simulink model "computed_torque_controller"  (R2020a)
settings: Solver=VariableStepAuto  StartTime=0.0  StopTime=50  RelTol=1e-3
model workspace (MAT data in the model file):
  kd = 0
  kp = 0
libraries: aerolibutil x4, sharedutil x2, simulink x1
settings Model: Creator=Sebas  LastModifiedBy=Sebas
settings SolverCC: ZeroCrossAlgorithm=Adaptive
settings DebuggingCC: MaskedZcDiagnostic=none  IgnoredZcDiagnostic=none

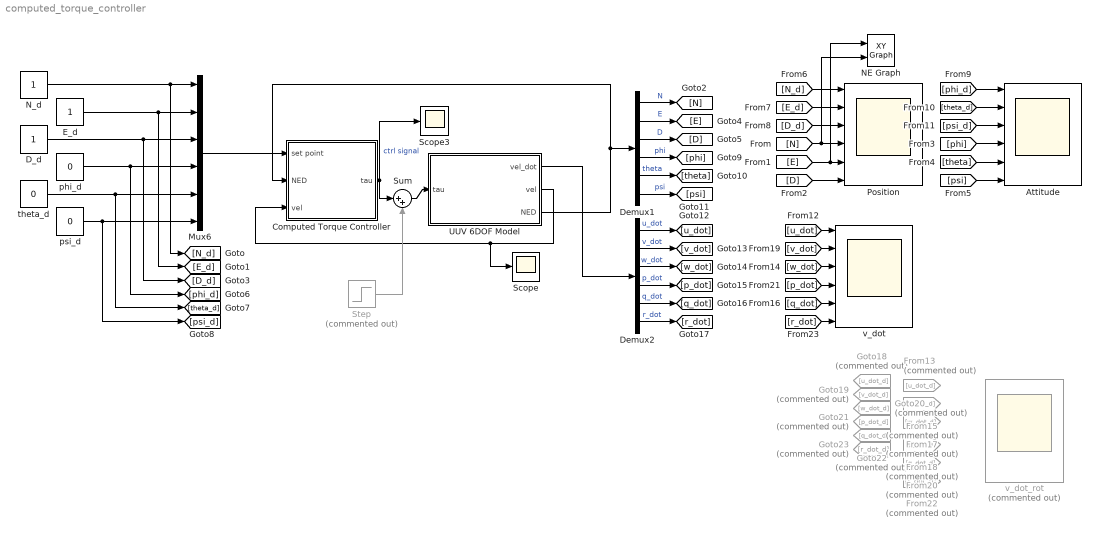
== system computed_torque_controller ==
  Attitude : Scope  NumInputPorts=6
  Computed Torque Controller : Subsystem
  D_d : Constant
  Demux1 : Demux  Outputs=6
  Demux2 : Demux  Outputs=6
  E_d : Constant
  From13 : From  Commented=on  GotoTag=u_dot_d
  From15 : From  Commented=on  GotoTag=v_dot_d
  From17 : From  Commented=on  GotoTag=w_dot_d
  From18 : From  Commented=on  GotoTag=p_dot_d
  From20 : From  Commented=on  GotoTag=q_dot_d
  From22 : From  Commented=on  GotoTag=r_dot_d
  Goto18 : Goto  Commented=on  GotoTag=u_dot_d
  Goto19 : Goto  Commented=on  GotoTag=v_dot_d
  Goto20 : Goto  Commented=on  GotoTag=w_dot_d
  Goto21 : Goto  Commented=on  GotoTag=p_dot_d
  Goto22 : Goto  Commented=on  GotoTag=q_dot_d
  Goto23 : Goto  Commented=on  GotoTag=r_dot_d
  Mux6 : Mux  Inputs=6
  NE Graph : simulink/Sinks/XY Graph  xmin=-1  xmax=5  ymin=-1  ymax=2  st=-1
  N_d : Constant
  Position : Scope  NumInputPorts=6
  Scope : Scope
  Scope3 : Scope
  Step : Step  Commented=on  Time=20  After=[30;30;30;5;5;5]  SampleTime=0
  Sum : Sum  Inputs=|++
  UUV 6DOF Model : Subsystem
  phi_d : Constant  Value=0
  psi_d : Constant  Value=0
  theta_d : Constant  Value=0
  v_dot : Scope  NumInputPorts=6
  v_dot_rot : Scope  Commented=on  NumInputPorts=6
  wires:
  UUV 6DOF Model/3(NED) -> Computed Torque Controller/2(NED), Demux1/1
  [N_d] -> Position/1
  [E_d] -> Position/2
  [D_d] -> Position/3
  [N] -> Position/4, NE Graph/2
  [D] -> Position/6
  [E] -> Position/5, NE Graph/1
  Demux1/1 -> [N]  "N"
  Demux1/2 -> [E]  "E"
  Demux1/3 -> [D]  "D"
  [phi_d] -> Attitude/1
  [phi] -> Attitude/4
  [psi_d] -> Attitude/3
  [theta] -> Attitude/5
  [psi] -> Attitude/6
  [theta_d] -> Attitude/2
  Demux1/4 -> [phi]  "phi"
  Demux1/5 -> [theta]  "theta"
  Demux1/6 -> [psi]  "psi"
  UUV 6DOF Model/2(vel) -> Computed Torque Controller/3(vel), Scope/1
  UUV 6DOF Model/1(vel_dot) -> Demux2/1
  [u_dot] -> v_dot/1
  [v_dot] -> v_dot/2
  [w_dot] -> v_dot/3
  [p_dot] -> v_dot/4
  [q_dot] -> v_dot/5
  [r_dot] -> v_dot/6
  Demux2/1 -> [u_dot]  "u_dot"
  Demux2/5 -> [q_dot]  "q_dot"
  Demux2/3 -> [w_dot]  "w_dot"
  Demux2/6 -> [r_dot]  "r_dot"
  Demux2/4 -> [p_dot]  "p_dot"
  Demux2/2 -> [v_dot]  "v_dot"
  D_d/1 -> Mux6/3, [D_d]
  theta_d/1 -> [theta_d], Mux6/5
  Mux6/1 -> Computed Torque Controller/1(set point)
  phi_d/1 -> Mux6/4, [phi_d]
  E_d/1 -> [E_d], Mux6/2
  N_d/1 -> [N_d], Mux6/1
  psi_d/1 -> [psi_d], Mux6/6
  Step/1 -> Sum/2
  Computed Torque Controller/1(tau) -> Sum/1, Scope3/1  "ctrl signal"
  Sum/1 -> UUV 6DOF Model/1(tau)

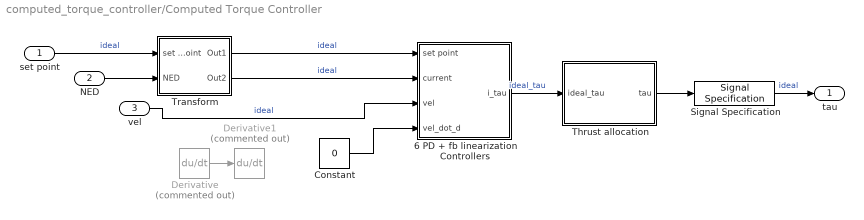
== system computed_torque_controller/Computed Torque Controller ==
  set point : Inport
  NED : Inport  Port=2
  vel : Inport  Port=3
  6 PD + fb linearization Controllers : Subsystem  mask(6 Degrees-of-freedom P-D Controller){surge_kd=0.35, surge_kp=0.7, sway_kd=0.7, sway_kp=0.6, heave_kd=0.2, heave_kp=0.7, roll_kd=1.3, roll_kp=10, pitch_kd=0.05, pitch_kp=0.2, yaw_kd=1.2, yaw_kp=3}
      mask prompts: surge_kd "Surge K derivative"; surge_kp "Surge K proportional"; sway_kd "Sway K derivative"; sway_kp "Sway K proportional"; heave_kd "Heave K derivative"; heave_kp "Heave K proportional"; roll_kd "Roll K derivative"; roll_kp "Roll K proportional"; pitch_kd "Pitch K derivative"; pitch_kp "Pitch K proportional"; yaw_kd "Yaw K derivative"; yaw_kp "Yaw K proportional"
      mask help: Implementation of 6 PD controllers for each degree of freedom
      mask DialogControl ParameterGroupVar Prompt: Gains
  Constant : Constant  Value=0
  Derivative : Derivative  Commented=on
  Derivative1 : Derivative  Commented=on
  Signal Specification : SignalSpecification  Dimensions=6
  Thrust allocation : Subsystem
  Transform : Subsystem
  tau : Outport
  wires:
  Transform/1(Out1) -> 6 PD + fb linearization Controllers/1(set point)  "ideal"
  NED/1 -> Transform/2(NED)
  Signal Specification/1 -> tau/1  "ideal"
  Transform/2(Out2) -> 6 PD + fb linearization Controllers/2(current)  "ideal"
  Thrust allocation/1(tau) -> Signal Specification/1
  6 PD + fb linearization Controllers/1(i_tau) -> Thrust allocation/1(ideal_tau)  "ideal_tau"
  vel/1 -> 6 PD + fb linearization Controllers/3(vel)  "ideal"
  set point/1 -> Transform/1(set point)  "ideal"
  Constant/1 -> 6 PD + fb linearization Controllers/4(vel_dot_d)
  Derivative/1 -> Derivative1/1

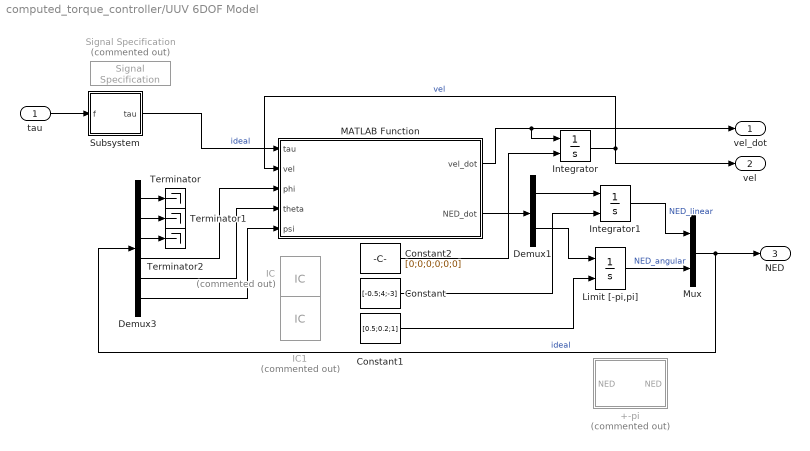
== system computed_torque_controller/UUV 6DOF Model ==
  tau : Inport
  +-pi : MATLAB Function  Commented=on  TreatAsAtomicUnit=on
  Constant : Constant  Value=[-0.5;4;-3]
  Constant1 : Constant  Value=[0.5;0.2;1]
  Constant2 : Constant  Value=[0;0;0;0;0;0]
  Demux1 : Demux  Outputs=2
  Demux3 : Demux  Outputs=6
  IC : InitialCondition  Commented=on  Value=[0;0;0;0;0;0]
  IC1 : InitialCondition  Commented=on  Value=[1;1;1;1;1;1]
  Integrator : Integrator  InitialConditionSource=external
  Integrator1 : Integrator  InitialConditionSource=external
  Limit [-pi,pi] : Integrator  InitialConditionSource=external  WrapState=on
  MATLAB Function : MATLAB Function  TreatAsAtomicUnit=on
  Mux : Mux  Inputs=2
  Signal Specification : SignalSpecification  Commented=on  Dimensions=6
  Subsystem : Subsystem
  Terminator : Terminator
  Terminator1 : Terminator
  Terminator2 : Terminator
  vel_dot : Outport
  vel : Outport  Port=2
  NED : Outport  Port=3
  wires:
  Constant/1 -> Integrator1/2
  Constant1/1 -> Limit [-pi,pi]/2
  Constant2/1 -> Integrator/2
  MATLAB Function/2(NED_dot) -> Demux1/1
  Demux1/1 -> Integrator1/1
  Demux1/2 -> Limit [-pi,pi]/1
  Limit [-pi,pi]/1 -> Mux/2  "NED_angular"
  tau/1 -> Subsystem/1(f)
  Subsystem/1(tau) -> MATLAB Function/1(tau)  "ideal"
  Demux3/3 -> Terminator2/1
  Demux3/1 -> Terminator/1
  Demux3/2 -> Terminator1/1
  Integrator1/1 -> Mux/1  "NED_linear"
  Demux3/6 -> MATLAB Function/5(psi)
  Demux3/5 -> MATLAB Function/4(theta)
  Demux3/4 -> MATLAB Function/3(phi)
  Integrator/1 -> MATLAB Function/2(vel), vel/1  "vel"
  MATLAB Function/1(vel_dot) -> Integrator/1, vel_dot/1
  Mux/1 -> NED/1, Demux3/1  "ideal"

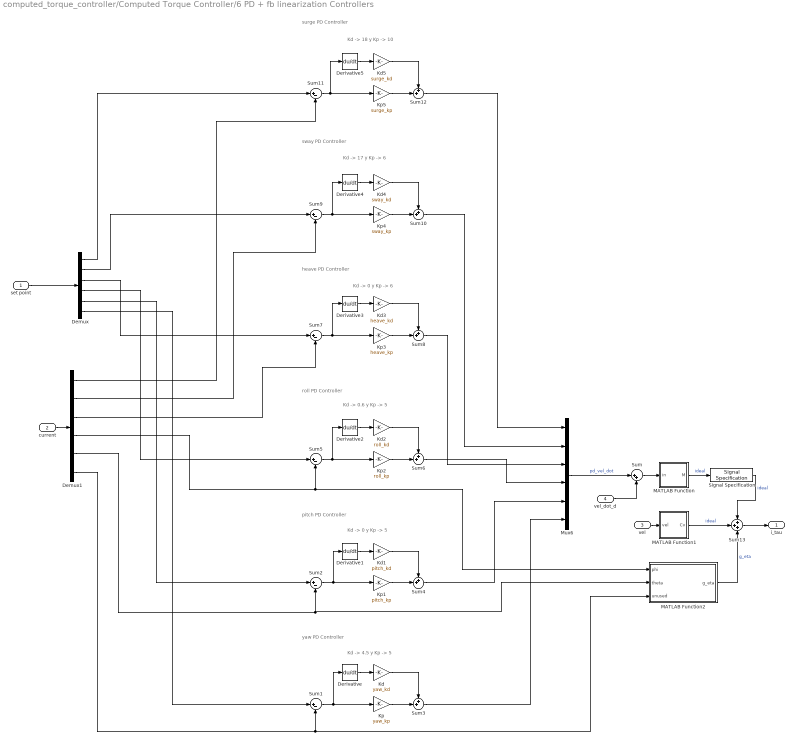
== system computed_torque_controller/Computed Torque Controller/6 PD + fb linearization Controllers ==
  note: surge PD Controller
  note: sway PD Controller
  note: heave PD Controller
  note: roll PD Controller
  note: pitch PD Controller
  note: yaw PD Controller
  note: Kd -> 4.5 y Kp -> 5
  note: Kd -> 0 y Kp -> 5
  note: Kd -> 0.6 y Kp -> 5
  note: Kd -> 0 y Kp -> 6
  note: Kd -> 17 y Kp -> 6
  note: Kd -> 18 y Kp -> 10
  set point : Inport
  current : Inport  Port=2
  vel : Inport  Port=3
  vel_dot_d : Inport  Port=4
  Demux : Demux  Outputs=6
  Demux1 : Demux  Outputs=6
  Derivative{,1..5} (6 alike) : Derivative
  Kd : Gain  Gain=yaw_kd
  Kd1 : Gain  Gain=pitch_kd
  Kd2 : Gain  Gain=roll_kd
  Kd3 : Gain  Gain=heave_kd
  Kd4 : Gain  Gain=sway_kd
  Kd5 : Gain  Gain=surge_kd
  Kp : Gain  Gain=yaw_kp
  Kp1 : Gain  Gain=pitch_kp
  Kp2 : Gain  Gain=roll_kp
  Kp3 : Gain  Gain=heave_kp
  Kp4 : Gain  Gain=sway_kp
  Kp5 : Gain  Gain=surge_kp
  MATLAB Function : MATLAB Function  TreatAsAtomicUnit=on
  MATLAB Function1 : MATLAB Function  TreatAsAtomicUnit=on
  MATLAB Function2 : MATLAB Function  TreatAsAtomicUnit=on
  Mux6 : Mux  Inputs=6
  Signal Specification : SignalSpecification  Dimensions=6
  Sum : Sum  Inputs=|++
  Sum{1..2,5,7,9,11} (6 alike) : Sum  Inputs=|+-
  Sum{3..4,6,8,10,12} (6 alike) : Sum  Inputs=++|
  Sum13 : Sum  Inputs=+++
  i_tau : Outport
  wires:
  Sum8/1 -> Mux6/3
  Sum4/1 -> Mux6/5
  Sum6/1 -> Mux6/4
  Sum3/1 -> Mux6/6
  Sum12/1 -> Mux6/1
  Sum10/1 -> Mux6/2
  Derivative/1 -> Kd/1
  Kp/1 -> Sum3/2
  Kd/1 -> Sum3/1
  Sum1/1 -> Derivative/1, Kp/1
  Sum2/1 -> Kp1/1, Derivative1/1
  Kd1/1 -> Sum4/1
  Kp1/1 -> Sum4/2
  Derivative1/1 -> Kd1/1
  Derivative2/1 -> Kd2/1
  Kp2/1 -> Sum6/2
  Kd2/1 -> Sum6/1
  Sum5/1 -> Derivative2/1, Kp2/1
  Derivative3/1 -> Kd3/1
  Kp3/1 -> Sum8/2
  Kd3/1 -> Sum8/1
  Sum7/1 -> Derivative3/1, Kp3/1
  Derivative4/1 -> Kd4/1
  Kp4/1 -> Sum10/2
  Kd4/1 -> Sum10/1
  Sum9/1 -> Derivative4/1, Kp4/1
  Derivative5/1 -> Kd5/1
  Kp5/1 -> Sum12/2
  Kd5/1 -> Sum12/1
  Sum11/1 -> Derivative5/1, Kp5/1
  current/1 -> Demux1/1
  Demux1/1 -> Sum11/2
  set point/1 -> Demux/1
  Demux/1 -> Sum11/1
  Demux/2 -> Sum9/1
  Demux1/2 -> Sum9/2
  Demux/3 -> Sum7/1
  Demux1/3 -> Sum7/2
  Demux/4 -> Sum5/1
  Demux1/4 -> MATLAB Function2/1(phi), Sum5/2
  Demux/5 -> Sum2/1
  Demux1/5 -> MATLAB Function2/2(theta), Sum2/2
  Demux/6 -> Sum1/1
  Demux1/6 -> MATLAB Function2/3(unused), Sum1/2
  Mux6/1 -> Sum/1  "pd_vel_dot"
  Sum/1 -> MATLAB Function/1(in)
  vel_dot_d/1 -> Sum/2
  Sum13/1 -> i_tau/1
  vel/1 -> MATLAB Function1/1(vel)
  MATLAB Function/1(M) -> Signal Specification/1  "ideal"
  MATLAB Function2/1(g_eta) -> Sum13/3  "g_eta"
  MATLAB Function1/1(Cv) -> Sum13/2  "ideal"
  Signal Specification/1 -> Sum13/1  "ideal"

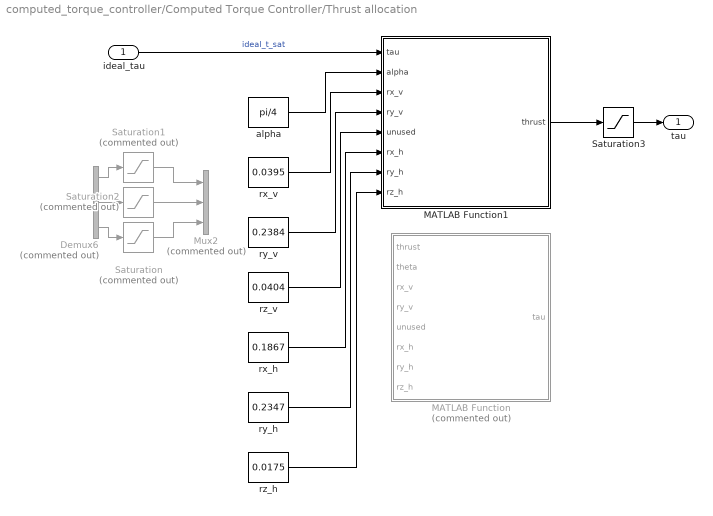
== system computed_torque_controller/Computed Torque Controller/Thrust allocation ==
  ideal_tau : Inport
  Demux6 : Demux  Commented=on  Outputs=3
  MATLAB Function : MATLAB Function  Commented=on  TreatAsAtomicUnit=on
  MATLAB Function1 : MATLAB Function  TreatAsAtomicUnit=on
  Mux2 : Mux  Commented=on  Inputs=3
  Saturation : Saturate  Commented=on  UpperLimit=70  LowerLimit=-70
  Saturation1 : Saturate  Commented=on  UpperLimit=100  LowerLimit=-100
  Saturation2 : Saturate  Commented=on  UpperLimit=100  LowerLimit=-100
  Saturation3 : Saturate  UpperLimit=35  LowerLimit=-35
  alpha : Constant  Value=pi/4
  rx_h : Constant  Value=0.1867
  rx_v : Constant  Value=0.0395
  ry_h : Constant  Value=0.2347
  ry_v : Constant  Value=0.2384
  rz_h : Constant  Value=0.0175
  rz_v : Constant  Value=0.0404
  tau : Outport
  wires:
  ideal_tau/1 -> MATLAB Function1/1(tau)  "ideal_t_sat"
  MATLAB Function1/1(thrust) -> Saturation3/1
  Saturation3/1 -> tau/1
  rx_v/1 -> MATLAB Function1/3(rx_v)
  alpha/1 -> MATLAB Function1/2(alpha)
  rx_h/1 -> MATLAB Function1/6(rx_h)
  ry_h/1 -> MATLAB Function1/7(ry_h)
  rz_h/1 -> MATLAB Function1/8(rz_h)
  ry_v/1 -> MATLAB Function1/4(ry_v)
  rz_v/1 -> MATLAB Function1/5(unused)
  Demux6/2 -> Saturation2/1
  Demux6/3 -> Saturation/1
  Saturation1/1 -> Mux2/1
  Saturation/1 -> Mux2/3
  Demux6/1 -> Saturation1/1
  Saturation2/1 -> Mux2/2

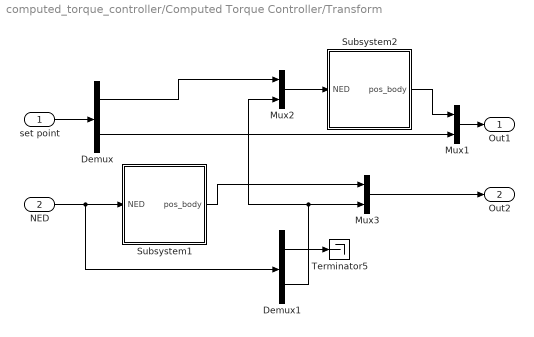
== system computed_torque_controller/Computed Torque Controller/Transform ==
  set point : Inport
  NED : Inport  Port=2
  Demux : Demux  Outputs=2
  Demux1 : Demux  Outputs=2
  Mux1 : Mux  Inputs=2
  Mux2 : Mux  Inputs=2
  Mux3 : Mux  Inputs=2
  Subsystem1 : Subsystem
  Subsystem2 : Subsystem
  Terminator5 : Terminator
  Out1 : Outport
  Out2 : Outport  Port=2
  wires:
  Demux/1 -> Mux2/1
  NED/1 -> Demux1/1, Subsystem1/1(NED)
  set point/1 -> Demux/1
  Demux/2 -> Mux1/2
  Subsystem2/1(pos_body) -> Mux1/1
  Demux1/1 -> Terminator5/1
  Subsystem1/1(pos_body) -> Mux3/1
  Demux1/2 -> Mux2/2, Mux3/2
  Mux2/1 -> Subsystem2/1(NED)
  Mux3/1 -> Out2/1
  Mux1/1 -> Out1/1

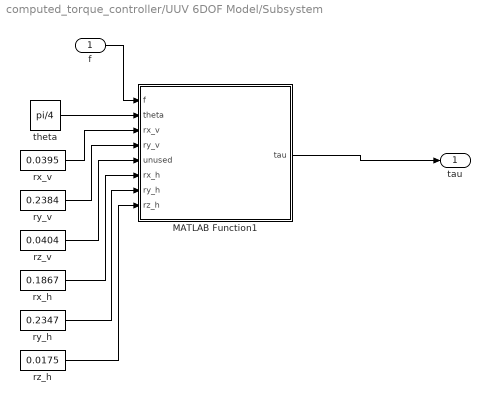
== system computed_torque_controller/UUV 6DOF Model/Subsystem ==
  f : Inport
  MATLAB Function1 : MATLAB Function  TreatAsAtomicUnit=on
  rx_h : Constant  Value=0.1867
  rx_v : Constant  Value=0.0395
  ry_h : Constant  Value=0.2347
  ry_v : Constant  Value=0.2384
  rz_h : Constant  Value=0.0175
  rz_v : Constant  Value=0.0404
  theta : Constant  Value=pi/4
  tau : Outport
  wires:
  rz_v/1 -> MATLAB Function1/5(unused)
  ry_h/1 -> MATLAB Function1/7(ry_h)
  f/1 -> MATLAB Function1/1(f)
  MATLAB Function1/1(tau) -> tau/1
  rx_h/1 -> MATLAB Function1/6(rx_h)
  theta/1 -> MATLAB Function1/2(theta)
  rx_v/1 -> MATLAB Function1/3(rx_v)
  rz_h/1 -> MATLAB Function1/8(rz_h)
  ry_v/1 -> MATLAB Function1/4(ry_v)

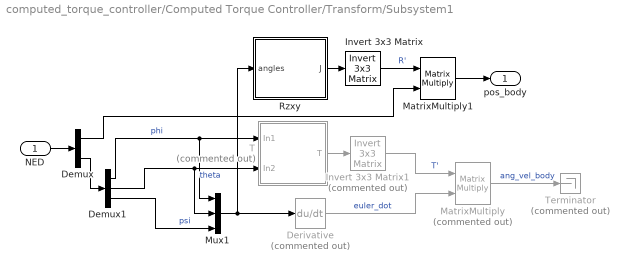
== system computed_torque_controller/Computed Torque Controller/Transform/Subsystem1 ==
  NED : Inport
  Demux : Demux  Outputs=2
  Demux1 : Demux  Outputs=3
  Derivative : Derivative  Commented=on
  Invert 3x3 Matrix : aerolibutil/Invert  3x3 Matrix
  Invert 3x3 Matrix1 : aerolibutil/Invert  3x3 Matrix  Commented=on
  MatrixMultiply : Product  Commented=on  Multiplication=Matrix(*)
  MatrixMultiply1 : Product  Multiplication=Matrix(*)
  Mux1 : Mux  Inputs=3
  Rzxy : Subsystem
  T : Subsystem  Commented=on
  Terminator : Terminator  Commented=on
  pos_body : Outport
  wires:
  Demux1/2 -> Mux1/2, T/2(In2)  "theta"
  Demux1/1 -> Mux1/1, T/1(In1)  "phi"
  Rzxy/1(J) -> Invert 3x3 Matrix/1
  Mux1/1 -> Derivative/1, Rzxy/1(angles)
  Derivative/1 -> MatrixMultiply/2  "euler_dot"
  Invert 3x3 Matrix1/1 -> MatrixMultiply/1  "T'"
  Demux1/3 -> Mux1/3  "psi"
  MatrixMultiply/1 -> Terminator/1  "ang_vel_body"
  T/1(T) -> Invert 3x3 Matrix1/1
  Invert 3x3 Matrix/1 -> MatrixMultiply1/1  "R'"
  MatrixMultiply1/1 -> pos_body/1
  NED/1 -> Demux/1
  Demux/2 -> Demux1/1
  Demux/1 -> MatrixMultiply1/2

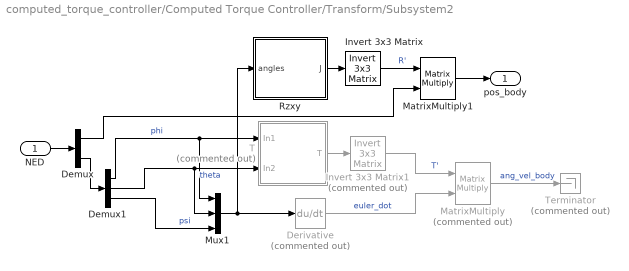
== system computed_torque_controller/Computed Torque Controller/Transform/Subsystem2 ==
  NED : Inport
  Demux : Demux  Outputs=2
  Demux1 : Demux  Outputs=3
  Derivative : Derivative  Commented=on
  Invert 3x3 Matrix : aerolibutil/Invert  3x3 Matrix
  Invert 3x3 Matrix1 : aerolibutil/Invert  3x3 Matrix  Commented=on
  MatrixMultiply : Product  Commented=on  Multiplication=Matrix(*)
  MatrixMultiply1 : Product  Multiplication=Matrix(*)
  Mux1 : Mux  Inputs=3
  Rzxy : Subsystem
  T : Subsystem  Commented=on
  Terminator : Terminator  Commented=on
  pos_body : Outport
  wires:
  Demux1/2 -> Mux1/2, T/2(In2)  "theta"
  Demux1/1 -> Mux1/1, T/1(In1)  "phi"
  Rzxy/1(J) -> Invert 3x3 Matrix/1
  Mux1/1 -> Derivative/1, Rzxy/1(angles)
  Derivative/1 -> MatrixMultiply/2  "euler_dot"
  Invert 3x3 Matrix1/1 -> MatrixMultiply/1  "T'"
  Demux1/3 -> Mux1/3  "psi"
  MatrixMultiply/1 -> Terminator/1  "ang_vel_body"
  T/1(T) -> Invert 3x3 Matrix1/1
  Invert 3x3 Matrix/1 -> MatrixMultiply1/1  "R'"
  MatrixMultiply1/1 -> pos_body/1
  NED/1 -> Demux/1
  Demux/2 -> Demux1/1
  Demux/1 -> MatrixMultiply1/2

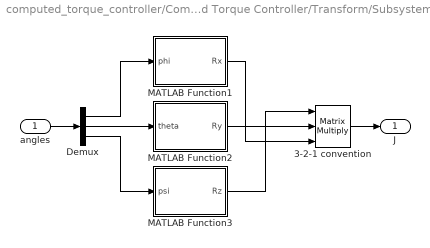
== system computed_torque_controller/Computed Torque Controller/Transform/Subsystem1/Rzxy ==
  angles : Inport
  3-2-1 convention : Product  Inputs=3  Multiplication=Matrix(*)
  Demux : Demux  Outputs=3
  MATLAB Function1 : MATLAB Function  TreatAsAtomicUnit=on
  MATLAB Function2 : MATLAB Function  TreatAsAtomicUnit=on
  MATLAB Function3 : MATLAB Function  TreatAsAtomicUnit=on
  J : Outport
  wires:
  Demux/1 -> MATLAB Function1/1(phi)
  MATLAB Function3/1(Rz) -> 3-2-1 convention/1
  MATLAB Function2/1(Ry) -> 3-2-1 convention/2
  Demux/3 -> MATLAB Function3/1(psi)
  MATLAB Function1/1(Rx) -> 3-2-1 convention/3
  3-2-1 convention/1 -> J/1
  angles/1 -> Demux/1
  Demux/2 -> MATLAB Function2/1(theta)

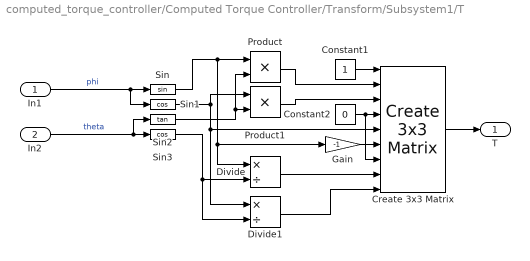
== system computed_torque_controller/Computed Torque Controller/Transform/Subsystem1/T ==
  In1 : Inport
  In2 : Inport  Port=2
  Constant1 : Constant
  Constant2 : Constant  Value=0
  Create 3x3 Matrix : sharedutil/Create 3x3 Matrix  aMode=aMode
      settings: SourceProductBaseCode=AE,PW,MT,VE,VP
  Divide : Product  Inputs=*/
  Divide1 : Product  Inputs=*/
  Gain : Gain  Gain=-1
  Product : Product
  Product1 : Product
  Sin : Trigonometry
  Sin1 : Trigonometry  Operator=cos
  Sin2 : Trigonometry  Operator=tan
  Sin3 : Trigonometry  Operator=cos
  T : Outport
  wires:
  Constant2/1 -> Create 3x3 Matrix/7, Create 3x3 Matrix/4
  Create 3x3 Matrix/1 -> T/1
  Gain/1 -> Create 3x3 Matrix/6
  Divide1/1 -> Create 3x3 Matrix/9
  Product/1 -> Create 3x3 Matrix/2
  Sin1/1 -> Divide1/1, Create 3x3 Matrix/5, Product1/1
  In1/1 -> Sin1/1, Sin/1  "phi"
  Sin2/1 -> Product/2, Product1/2
  Divide/1 -> Create 3x3 Matrix/8
  Product1/1 -> Create 3x3 Matrix/3
  Sin3/1 -> Divide1/2, Divide/2
  In2/1 -> Sin2/1, Sin3/1  "theta"
  Sin/1 -> Gain/1, Divide/1, Product/1
  Constant1/1 -> Create 3x3 Matrix/1

== system computed_torque_controller/Computed Torque Controller/Transform/Subsystem2/Rzxy ==
  angles : Inport
  3-2-1 convention : Product  Inputs=3  Multiplication=Matrix(*)
  Demux : Demux  Outputs=3
  MATLAB Function1 : MATLAB Function  TreatAsAtomicUnit=on
  MATLAB Function2 : MATLAB Function  TreatAsAtomicUnit=on
  MATLAB Function3 : MATLAB Function  TreatAsAtomicUnit=on
  J : Outport
  wires:
  Demux/1 -> MATLAB Function1/1(phi)
  MATLAB Function3/1(Rz) -> 3-2-1 convention/1
  MATLAB Function2/1(Ry) -> 3-2-1 convention/2
  Demux/3 -> MATLAB Function3/1(psi)
  MATLAB Function1/1(Rx) -> 3-2-1 convention/3
  3-2-1 convention/1 -> J/1
  angles/1 -> Demux/1
  Demux/2 -> MATLAB Function2/1(theta)

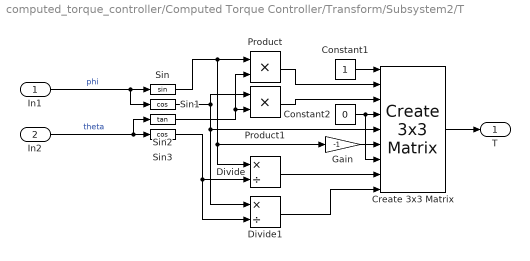
== system computed_torque_controller/Computed Torque Controller/Transform/Subsystem2/T ==
  In1 : Inport
  In2 : Inport  Port=2
  Constant1 : Constant
  Constant2 : Constant  Value=0
  Create 3x3 Matrix : sharedutil/Create 3x3 Matrix  aMode=aMode
      settings: SourceProductBaseCode=AE,PW,MT,VE,VP
  Divide : Product  Inputs=*/
  Divide1 : Product  Inputs=*/
  Gain : Gain  Gain=-1
  Product : Product
  Product1 : Product
  Sin : Trigonometry
  Sin1 : Trigonometry  Operator=cos
  Sin2 : Trigonometry  Operator=tan
  Sin3 : Trigonometry  Operator=cos
  T : Outport
  wires:
  Constant2/1 -> Create 3x3 Matrix/7, Create 3x3 Matrix/4
  Create 3x3 Matrix/1 -> T/1
  Gain/1 -> Create 3x3 Matrix/6
  Divide1/1 -> Create 3x3 Matrix/9
  Product/1 -> Create 3x3 Matrix/2
  Sin1/1 -> Divide1/1, Create 3x3 Matrix/5, Product1/1
  In1/1 -> Sin1/1, Sin/1  "phi"
  Sin2/1 -> Product/2, Product1/2
  Divide/1 -> Create 3x3 Matrix/8
  Product1/1 -> Create 3x3 Matrix/3
  Sin3/1 -> Divide1/2, Divide/2
  In2/1 -> Sin2/1, Sin3/1  "theta"
  Sin/1 -> Gain/1, Divide/1, Product/1
  Constant1/1 -> Create 3x3 Matrix/1

== matlab function computed_torque_controller/Computed Torque Controller/Transform/Subsystem1/Rzxy/MATLAB Function2 ==
  data: theta input; Ry output
function Ry = Ry(theta)
Ry = [ cos(theta) 0 sin(theta);
       0          1     0 ;
       -sin(theta) 0 cos(theta); ];

== matlab function computed_torque_controller/Computed Torque Controller/Transform/Subsystem1/Rzxy/MATLAB Function3 ==
  data: psi input; Rz output
function Rz = Rz(psi)
Rz = [ cos(psi) -sin(psi) 0;
       sin(psi) cos(psi)  0;
       0        0         1];

== matlab function computed_torque_controller/Computed Torque Controller/Thrust allocation/MATLAB Function1 ==
  data: tau input; thrust output; alpha input; rx_v input; ry_v input; unused input; rx_h input; ry_h input; rz_h input
function thrust = thrust_allocation(tau, alpha, rx_v, ry_v, ~, rx_h, ry_h, rz_h)
% Mapping matrix
T = [cos(alpha) cos(alpha) -cos(alpha) -cos(alpha) 0 0;
     -sin(alpha) sin(alpha) -sin(alpha) sin(alpha) 0 0;
     0 0 0 0 -1 -1;
     -sin(alpha)*rz_h sin(alpha)*rz_h -sin(alpha)*rz_h sin(alpha)*rz_h -ry_v ry_v;
     -cos(alpha)*rz_h -cos(alpha)*rz_h cos(alpha)*rz_h cos(alpha)*rz_h -rx_v rx_v;
     -(rx_h*sin(alpha)+ry_h*cos(alpha)) (rx_h*sin(alpha)+ry_h*cos(alpha)) (rx_h*sin(alpha)+ry_h*cos(alpha)) -(rx_h*sin(alpha)+ry_h*cos(alpha)) 0 0
    ];
% Control input with Moore–Penrose pseudo-inverse
t = pinv(T)*tau;
thrust = t;

== matlab function computed_torque_controller/Computed Torque Controller/6 PD + fb linearization Controllers/MATLAB Function ==
  data: M output; in input
function M = M(in)
% Skew symmetric matrix
S = @(s) [0    -s(3) s(2);
          s(3) 0     -s(1);
          -s(2) s(1)  0    ];  

% Vehicle parameters
m = 24;

r_g = [0 0 0].';    % Distance from origin to center of mass
I_g = [0.900121387  -0.000186482 0.0072251;
       -0.000186482 1.754494427  0.020319615;
       0.0072251    0.020319615  1.43389     ]; % Rigid-body inertia matrix

% Rigid-Body Inertia Matrix
M_rb = [ m*eye(3)    -m*S(r_g);
         m*S(r_g)         I_g ];

% Added mass matrix
M_a = diag([16.8374 20.2748 35.3180 0.2165 0.6869 0.6157]);

% Mass matrix
M = (M_rb + M_a)*in;

== matlab function computed_torque_controller/Computed Torque Controller/6 PD + fb linearization Controllers/MATLAB Function1 ==
  data: Cv output; vel input
function Cv = C(vel)
v = [0;0;0;0;0;0];
% Skew symmetric matrix
S = @(s) [0    -s(3) s(2);
          s(3) 0     -s(1);
          -s(2) s(1)  0    ];  

% Vehicle parameters
m = 24;

r_g = [0 0 0].';    % Distance from origin to center of mass
I_g = [0.900121387  -0.000186482 0.0072251;
       -0.000186482 1.754494427  0.020319615;
       0.0072251    0.020319615  1.43389     ]; % Rigid-body inertia matrix

% Added mass matrix
M_a = diag([16.8374 20.2748 35.3180 0.2165 0.6869 0.6157]);

%------------ UUV dynamic model parametrization ----------------%
% Rigid-body Coriolis-centripetal Matrix
C_rb = [ zeros(3)             -m*S(vel(1:3))-m*S(vel(4:6))*S(r_g);
        -m*S(vel(1:3))+m*S(r_g)*S(vel(4:6))            -S(I_g*vel(4:6))];

% Coreolis added mass matrix 
C_a = [ 0 0 0   0 -M_a(3,3)*vel(3) M_a(2,2)*vel(2) ;
        0 0 0   M_a(3,3)*vel(3) 0 -M_a(1,1)*vel(1) ;
        0 0 0  -M_a(2,2)*vel(2) M_a(1,1)*vel(1) 0  ;
        0 -M_a(3,3)*vel(3) M_a(2,2)*vel(2)  0 -M_a(6,6)*vel(6) M_a(5,5)*vel(5) ;
        M_a(3,3)*vel(3) 0 -M_a(1,1)*vel(1)  M_a(6,6)*vel(6) 0 -M_a(4,4)*vel(4) ;
       -M_a(2,2)*vel(2) M_a(1,1)*vel(1) 0   -M_a(5,5)*vel(5) M_a(4,4)*vel(4) 0  ];
v = vel;
% Coreolis matrix
C = C_rb + C_a;
Cv = C*v;

== matlab function computed_torque_controller/Computed Torque Controller/6 PD + fb linearization Controllers/MATLAB Function2 ==
  data: phi input; theta input; g_eta output; unused input
function g_eta = g_eta(phi, theta, ~)
%Fossen (2011): According to (2.2), the sign of the restoring forces and moments fbi 
%and mbi = rbi × fbi , i ∈ {g, b}, must be changed when moving these terms to the 
%left-hand side of (2.2) that is the vector g(η). Pag 60 Handbook of ...

r_g = [0 0 0].';    % Distance from origin to center of mass
r_b = [0 0 -0.10726].';    % Distance from origin to center of buoyancy
m = 24;
W = m*9.81;
B = W*1.005; 
% Restoring forces
g_eta = [ (W-B)*sin(theta);
          -(W-B)*cos(theta)*sin(phi);
          -(W-B)*cos(theta)*cos(phi);
          -(r_g(2)*W-r_b(2)*B)*cos(theta)*cos(phi) + (r_g(3)*W-r_b(3)*B)*cos(theta)*sin(phi);
           (r_g(3)*W-r_b(3)*B)*sin(theta)             + (r_g(1)*W-r_b(1)*B)*cos(theta)*cos(phi)
          -(r_g(1)*W-r_b(1)*B)*cos(theta)*sin(phi) - (r_g(2)*W-r_b(2)*B)*sin(theta)          ];

== matlab function computed_torque_controller/Computed Torque Controller/Transform/Subsystem2/Rzxy/MATLAB Function1 ==
  data: phi input; Rx output
function Rx = Rx(phi)
Rx = [ 1 0 0;
       0 cos(phi) -sin(phi);
       0 sin(phi) cos(phi); ];

== matlab function computed_torque_controller/UUV 6DOF Model/+-pi ==
  data: NED input; NED output
function NED = check_angles(NED)
% Correct
if abs(NED(4)) > pi 
    NED(4) = (NED(4)/abs(NED(4)))*(abs(NED(4))-2*pi);
end
if abs(NED(5)) > pi 
    NED(5) = (NED(5)/abs(NED(5)))*(abs(NED(5))-2*pi);
end
if abs(NED(6)) > pi
    NED(6) = (NED(6)/abs(NED(6)))*(abs(NED(6))-2*pi);
    disp((NED(6)/abs(NED(6)))*(abs(NED(6))-2*pi))
end

== matlab function computed_torque_controller/Computed Torque Controller/Thrust allocation/MATLAB Function ==
  data: thrust input; tau output; theta input; rx_v input; ry_v input; unused input; rx_h input; ry_h input; rz_h input
function tau = thrust_conversion(thrust, theta, rx_v, ry_v, ~, rx_h, ry_h, rz_h)
% Errores numericos. El input esta saturado a [100,-100], y estas salidas
% dan valores muchisimo mayores a 35 N c/u
tau = [0 0 0 0 0 0].';
% For surge
s_val = thrust(1)/cos(theta)/4;
tau(1) = tau(1)+s_val;
tau(2) = tau(2)+s_val;
tau(3) = tau(3)-s_val;
tau(4) = tau(4)-s_val;

% For sway
sw_val = thrust(2)/sin(theta)/4;
tau(1) = tau(1)-sw_val;
tau(2) = tau(2)+sw_val;
tau(3) = tau(3)-sw_val;
tau(4) = tau(4)+sw_val;

% For heave
tau(5) = tau(5)+(-thrust(3)/2);
tau(6) = tau(6)+(-thrust(3)/2);

% For yaw
y_val = thrust(6)/(rx_h*sin(theta)+ry_h*cos(theta))/4;
tau(1) = tau(1)-y_val;
tau(2) = tau(2)+y_val;
tau(3) = tau(3)+y_val;
tau(4) = tau(4)-y_val;

% K and M come as zero
% For K
if  thrust(4)~= 0
    %disp("K")
    k_val = (thrust(4)-(-tau(1)+tau(2)-tau(3)+tau(4))*sin(theta)*rz_h)/(2*ry_v);
    tau(5) = tau(5)-k_val;
    tau(6) = tau(6)+k_val;
end

% For M
if thrust(5) ~= 0
    %disp("M")
    M_val = (thrust(5)-(-tau(1)-tau(2)+tau(3)+tau(4))*cos(theta)*rz_h)/(2*rx_v);
    tau(5) = tau(5)-M_val;
    tau(6) = tau(6)+M_val;
end
disp(tau)

== matlab function computed_torque_controller/UUV 6DOF Model/MATLAB Function ==
  data: vel_dot output; tau input; vel input; phi input; theta input; NED_dot output; psi input
function [vel_dot,NED_dot]= UUV_forward_dynamics(tau,vel,phi,theta,psi)
% Skew symmetric matrix
S = @(s) [0    -s(3) s(2);
          s(3) 0     -s(1);
          -s(2) s(1)  0    ];  

% Vehicle parameters
m = 24;
vol = 0.02306187;
W = m*9.81;
B = W*1.005; %1000*9.81*vol;

r_g = [0 0 0].';    % Distance from origin to center of mass
r_b = [0 0 -0.10726].';    % Distance from origin to center of buoyancy
I_g = [0.900121387  -0.000186482 0.0072251;
       -0.000186482 1.754494427  0.020319615;
       0.0072251    0.020319615  1.43389     ]; % Rigid-body inertia matrix

% Rigid-Body Inertia Matrix
M_rb = [ m*eye(3)    -m*S(r_g);
         m*S(r_g)         I_g ];

% Added mass matrix
M_a = diag([16.8374 20.2748 35.3180 0.2165 0.6869 0.6157]);

% Mass matrix
M = M_rb + M_a;

% Linear damping coefficients
X_u = -0.3431;
Y_v = 0.0518;
Z_w = -0.5841;
K_p = 0.0064;
M_q = 0.04;
N_r = -0.1063;

D_lin = -diag([X_u Y_v Z_w K_p M_q N_r]);

% Cuadratic damping coefficients
X_uu = -111.7397;
Y_vv = -44.4058;
Z_ww = -157.1951;
K_pp = -0.4634;
M_qq = -0.2902;
N_rr = -2.2897;

%------------ UUV dynamic model parametrization ----------------%
% Rigid-body Coriolis-centripetal Matrix
C_rb = [ zeros(3)             -m*S(vel(1:3))-m*S(vel(4:6))*S(r_g);
        -m*S(vel(1:3))+m*S(r_g)*S(vel(4:6))            -S(I_g*vel(4:6))];

% Coreolis added mass matrix 
C_a = [ 0 0 0   0 -M_a(3,3)*vel(3) M_a(2,2)*vel(2) ;
        0 0 0   M_a(3,3)*vel(3) 0 -M_a(1,1)*vel(1) ;
        0 0 0  -M_a(2,2)*vel(2) M_a(1,1)*vel(1) 0  ;
        0 -M_a(3,3)*vel(3) M_a(2,2)*vel(2)  0 -M_a(6,6)*vel(6) M_a(5,5)*vel(5) ;
        M_a(3,3)*vel(3) 0 -M_a(1,1)*vel(1)  M_a(6,6)*vel(6) 0 -M_a(4,4)*vel(4) ;
       -M_a(2,2)*vel(2) M_a(1,1)*vel(1) 0   -M_a(5,5)*vel(5) M_a(4,4)*vel(4) 0  ];

% Coreolis matrix
C = C_rb + C_a;

% Restoring forces
g_eta = [ (W-B)*sin(theta);
          -(W-B)*cos(theta)*sin(phi);
          -(W-B)*cos(theta)*cos(phi);
          -(r_g(2)*W-r_b(2)*B)*cos(theta)*cos(phi) + (r_g(3)*W-r_b(3)*B)*cos(theta)*sin(phi);
           (r_g(3)*W-r_b(3)*B)*sin(theta)             + (r_g(1)*W-r_b(1)*B)*cos(theta)*cos(phi)
          -(r_g(1)*W-r_b(1)*B)*cos(theta)*sin(phi) - (r_g(2)*W-r_b(2)*B)*sin(theta)          ];

% Cuadratic Damping matrix
D_cuad = -diag([X_uu*abs(vel(1)) Y_vv*abs(vel(2)) Z_ww*abs(vel(3)) ...
               K_pp*abs(vel(4)) M_qq*abs(vel(5)) N_rr*abs(vel(6))]);

%Damping matrix
Damp = D_lin + D_cuad;

NED_dot = [0;0;0;0;0;0];
% Linear velocities in NED / For a zxy rotation sequence
NED_dot(1) = vel(1)*cos(psi)*cos(theta) + vel(2)*[cos(psi)*sin(theta)*sin(phi)... 
    - sin(psi)*cos(phi)] + vel(3)*[sin(psi)*sin(phi)... 
    + cos(psi)*cos(phi)*sin(theta)];

NED_dot(2) = vel(1)*sin(psi)*cos(theta) + vel(2)*[cos(psi)*cos(phi)... 
    + sin(phi)*sin(theta)*sin(psi)]+ vel(3)*[sin(theta)*sin(psi)*cos(phi)... 
    - cos(psi)*sin(phi)];

NED_dot(3) = -vel(1)*sin(theta) + vel(2)*cos(theta)*sin(phi) + vel(3)*cos(theta)*cos(phi);

%Angular velocities in NED
NED_dot(4) = vel(4) + vel(5)*sin(phi)*tan(theta) + vel(6)*cos(phi)*tan(theta);

NED_dot(5) = vel(5)*cos(phi) - vel(6)*sin(phi);

NED_dot(6) = vel(5)*(sin(phi)/cos(theta)) + vel(6)*(cos(phi)/cos(theta));

vel_dot = M\(tau-(C*vel)-(Damp*vel)-g_eta);

== matlab function computed_torque_controller/UUV 6DOF Model/Subsystem/MATLAB Function1 ==
  data: tau output; f input; theta input; rx_v input; ry_v input; unused input; rx_h input; ry_h input; rz_h input
function tau = tau_conversion(f, theta, rx_v, ry_v, ~, rx_h, ry_h, rz_h)
tau = [0 0 0 0 0 0].';
tau(1) = (f(1)+f(2)-f(3)-f(4))*cos(theta);
tau(2) = (-f(1)+f(2)-f(3)+f(4))*sin(theta);
tau(3) = -(f(5)+f(6));
tau(4) = (f(6)-f(5))*ry_v + (-f(1)+f(2)-f(3)+f(4))*sin(theta)*rz_h;
tau(5) = (f(6)-f(5))*rx_v + (-f(1)-f(2)+f(3)+f(4))*cos(theta)*rz_h;
tau(6) = (-f(1)+f(2)+f(3)-f(4))*(rx_h*sin(theta)+ry_h*cos(theta));

== matlab function computed_torque_controller/Computed Torque Controller/Transform/Subsystem2/Rzxy/MATLAB Function2 ==
  data: theta input; Ry output
function Ry = Ry(theta)
Ry = [ cos(theta) 0 sin(theta);
       0          1     0 ;
       -sin(theta) 0 cos(theta); ];

== matlab function computed_torque_controller/Computed Torque Controller/Transform/Subsystem2/Rzxy/MATLAB Function3 ==
  data: psi input; Rz output
function Rz = Rz(psi)
Rz = [ cos(psi) -sin(psi) 0;
       sin(psi) cos(psi)  0;
       0        0         1];

== matlab function computed_torque_controller/Computed Torque Controller/Transform/Subsystem1/Rzxy/MATLAB Function1 ==
  data: phi input; Rx output
function Rx = Rx(phi)
Rx = [ 1 0 0;
       0 cos(phi) -sin(phi);
       0 sin(phi) cos(phi); ];
